simulink model "test4"  (R2021a)
settings: Solver=VariableStepAuto  StartTime=0.0  StopTime=20  RelTol=1e-1
undefined symbols (not defined in the file): B_EMB, C1, C_EMB, D_EMB, f, i_EMB, JL, JM, Jm_EMB, K1, N_EMB, rb_EMB, s_EMB, sigbuilder_block, Tc_EMB, Ts_EMB, ub_EMB
libraries: powerlib_extras x9, spsDCVoltageSourceLib x5, spsPermanentMagnetSynchronousMachineLib x5, spsUniversalBridgeLib x5, spspowerguiLib x5, spsVoltageMeasurementLib x4, pid_lib x4, simulink x3, dsparch4 x2, instrumentlib x2, Solver_SF x1
(part 3 of 3)

== matlab function test4/驱动电机模型4/2_vector_MPC_control1 ==
  settings: updateMethod=DISCRETE
  data: clock input; i_q_k input; i_d_k input; theta_e_r input; flux input; Ld input; Lq input; sa output; sb output; sc output; dtheta_e input; Te_k input; Te_ref input; phi_s_ref input
function [sa, sb, sc ] = fcn(clock, i_q_k, i_d_k, theta_e_r, flux, Ld, Lq, dtheta_e, Te_k, Te_ref, phi_s_ref)
%% 参数初始化
Ts = 0.0001;
cost = inf;
vdc = 400; % 定子电压
Rs = 0.01; % 电阻
pn = 4;
%% 获取控制周期内的相对时间
persistent time_start;
if isempty(time_start)
    time_start = clock;
end
time_relative = clock-time_start;
if time_relative >= Ts-1e-12
    time_start = clock;
    time_relative = 0;
end

%% 计算参考电压矢量
% % 无差拍控制下的phi_alpha\phi_beta
% ud_k = 0;
% ud_k = 0;
% i_d_k1 = (1-Rs*Ts/Ld)*i_d_k+Ts/Ld*(ud_k+dtheta_e*Lq*i_q_k);
% i_q_k1 = (1-Rs*Ts/Ld)*i_q_k+Ts/Ld*(uq_k-dtheta_e*Ld*i_d_k + dtheta_e*flux)

phi_dk = Ld*i_d_k +flux;
phi_qk = Lq*i_q_k;
X1 = phi_dk+dtheta_e*phi_qk*Ts;
B = ((2*Lq)/(3*pn*flux))*(Te_ref-Te_k) + (Rs*Ts*phi_qk)/Lq + dtheta_e*Ts*phi_dk;
X2 = B^2 + 2*B*(phi_qk-dtheta_e*phi_dk*Ts)+(1+dtheta_e^2*Ts^2)*(phi_dk^2+phi_qk^2) - phi_s_ref^2;
radicand = X1^2 - X2;
radicand = max(radicand, 1e-9);  % 限制最小值为1e-9，避免sqrt报错

ud_ref1 = (-X1 + sqrt(radicand)) / Ts;
ud_ref2 = (-X1 - sqrt(radicand)) / Ts;
% 选择幅值较小的解
if abs(ud_ref1) <= abs(ud_ref2)
    ud_ref = ud_ref1;
else
    ud_ref = ud_ref2;
end


uq_ref = B/Ts;
u_alpha_ref = cos(theta_e_r)*ud_ref - sin(theta_e_r)*uq_ref;
u_beta_ref = sin(theta_e_r)*ud_ref + cos(theta_e_r)*uq_ref;
theta_u_ref = atan2(u_beta_ref, u_alpha_ref);
if theta_u_ref<0
    theta_u_ref=theta_u_ref+2*pi;
end
%% 计算选择矢量
% 选择第一电压矢量
theta_norm_rel = theta_u_ref + pi/6;
if theta_norm_rel>2*pi
    theta_norm_rel=theta_norm_rel-2*pi;
end

sector = floor(theta_norm_rel / (pi/3)) + 1;
% 处理边界情况（刚好在扇区边界时归为当前扇区）
if sector == 7
    sector = 1;
end
voltage_vectors = [
    0 0 0;  % 0矢量V0
    1 0 0;  % 扇区1第一矢量V1
    1 1 0;  % 扇区2第一矢量V2
    0 1 0;  % 扇区3第一矢量V3
    0 1 1;  % 扇区4第一矢量V4
    0 0 1;  % 扇区5第一矢量V5
    1 0 1;  % 扇区6第一矢量V6
    1 1 1]; % 0矢量V7
% 选择当前扇区的第一电压矢量
first_vector = voltage_vectors(sector+1, :);
ua1 = first_vector(1)*vdc;
ub1 = first_vector(2)*vdc;
uc1 = first_vector(3)*vdc;
un1 = (ua1+ub1+uc1)/3;
u_an1 = ua1 - un1;
u_bn1 = ub1 - un1;
u_cn1 = uc1 - un1;
u_alpha_first = 2/3*(u_an1 - 1/2*u_bn1 - 1/2*u_cn1);
u_beta_first = 2/3*(sqrt(3)/2*u_bn1 - sqrt(3)/2*u_cn1);
% 选择第二电压矢量
% 开关次数约束
adjacent_sectors = {
    [7, 3, 1];  % 扇区1（V1）的相邻矢量：扇区2（V2）、扇区6（V6）
    [2, 4, 8];  % 扇区2（V2）的相邻矢量：扇区1（V1）、扇区3（V3）
    [3, 5, 1];  % 扇区3（V3）的相邻矢量：扇区2（V2）、扇区4（V4）
    [4, 6, 8];  % 扇区4（V4）的相邻矢量：扇区3（V3）、扇区5（V5）
    [5, 7, 1];  % 扇区5（V5）的相邻矢量：扇区4（V4）、扇区6（V6）
    [6, 2, 8]   % 扇区6（V6）的相邻矢量：扇区5（V5）、扇区1（V1）
    };
allowed_second_sectors = adjacent_sectors{sector};  % 允许的第二矢量sector

second_state = allowed_second_sectors(1);
for i = allowed_second_sectors
    second_vector = voltage_vectors(i,:);
    ua2 = second_vector(1)*vdc;
    ub2 = second_vector(2)*vdc;
    uc2 = second_vector(3)*vdc;
    un2 = (ua2+ub2+uc2)/3;
    u_an2 = ua2 - un2;
    u_bn2 = ub2 - un2;
    u_cn2 = uc2 - un2;
    u_alpha_second = 2/3*(u_an2 - 1/2*u_bn2 - 1/2*u_cn2);
    u_beta_second = 2/3*(sqrt(3)/2*u_bn2 - sqrt(3)/2*u_cn2);
    J = sqrt((u_alpha_ref-u_alpha_second)^2 + (u_beta_ref-u_beta_second)^2);
    if J<cost
        cost = J;
        second_state = i;
    end
    
end

second_vector = voltage_vectors(second_state, :);



%% 计算矢量作用时间
% αβ坐标系下参考电压矢量
% u_alpha_ref = Rs * i_alpha_k + (phi_alpha_k1 - phi_alpha_k)/Ts;
% u_beta_ref = Rs * i_beta_k + (phi_beta_k1 - phi_beta_k)/Ts;

% αβ坐标系下第一电压矢量
% u_alpha_first = 2/3*(u_an1 - 1/2*u_bn1 - 1/2*u_cn1);
% u_beta_first = 2/3*(sqrt(3)/2*u_bn1 - sqrt(3)/2*u_cn1);

% αβ坐标系下第二电压矢量
% u_alpha_second = 2/3*(u_an - 1/2*u_bn - 1/2*u_cn);
% u_beta_second = 2/3*(sqrt(3)/2*u_bn - sqrt(3)/2*u_cn);
num1 = (u_alpha_ref-u_alpha_second)*(u_alpha_first-u_alpha_second)+(u_beta_ref-u_beta_second)*(u_beta_first-u_beta_second);
num2 = (u_alpha_second-u_alpha_first)^2+(u_beta_second-u_beta_first)^2;
% num1 = u_alpha_ref*u_alpha_first + u_beta_ref*u_beta_first;
% num2 = u_alpha_ref^2+u_beta_ref^2;

t_1opt = num1/num2;

if t_1opt>1 
    t_1opt = 1;
end
if t_1opt<0
    t_1opt = 0;
end
% t_2opt = Ts - t_1opt;



%% 输出矢量
if time_relative < t_1opt*Ts-1e-12
%if time_relative < 2*Ts-1e-12
    sa = first_vector(1);
    sb = first_vector(2);
    sc = first_vector(3);

else
    sa = second_vector(1);
    sb = second_vector(2);
    sc = second_vector(3);    

end

== matlab function test4/驱动电机模型4/MTPA ==
  data: Te input; phi_s_ref output; Pn input; flux input; Ld input; Lq input; ita_ref output
function [phi_s_ref, ita_ref] = fcn(Te, Pn, flux, Ld, Lq)
%% MPTA原则计算phi_s_ref和ita_ref
% 对于表贴式PMSM (Ld = Lq)，MPTA条件就是id=0控制

% 计算q轴电流参考（id_ref = 0）
iq_ref = Te / (1.5 * Pn * flux);

% 计算定子磁链参考值
% phi_d = flux + Ld * id_ref = flux
% phi_q = Lq * iq_ref
phi_d_ref = flux;      % id=0
phi_q_ref = Lq * iq_ref;

phi_s_ref = sqrt(phi_d_ref^2 + phi_q_ref^2);

% 计算定子磁链参考角度
if abs(Te) < 1e-6
    ita_ref = 0;  % 零转矩时角度为0
else
    ita_ref = atan2(phi_q_ref, phi_d_ref);
end

% 确保角度在合理范围内
ita_ref = real(ita_ref);  % 避免复数
end

== matlab function test4/驱动电机模型4/phi_s_k ==
  data: id_k input; phi_s_k output; iq_k input; flux input; Ld input; Lq input; ita_k output
function [phi_s_k,ita_k]  = fcn(id_k,iq_k,flux,Ld,Lq)
phi_q_k = Lq*iq_k;
phi_d_k = Ld*id_k + flux;
phi_s_k = sqrt(phi_q_k^2+phi_d_k^2);
ita_k = atan2(phi_q_k, phi_d_k);

end

== matlab function test4/驱动电机模型1/2_vector_MPC_control1 ==
  settings: updateMethod=DISCRETE
  data: clock input; i_q_k input; i_d_k input; theta_e_r input; sa output; sb output; sc output; flux input; Ld input; Lq input; dtheta_e input; Te_k input; Te_ref input; phi_s_ref input
function [sa, sb, sc ] = fcn(clock, i_q_k, i_d_k, theta_e_r, flux, Ld, Lq, dtheta_e, Te_k, Te_ref, phi_s_ref)
%% 参数初始化
Ts = 0.0001;
cost = inf;
vdc = 400; % 定子电压
Rs = 0.11; % 电阻
pn = 4;
%% 获取控制周期内的相对时间
persistent time_start;
if isempty(time_start)
    time_start = clock;
end
time_relative = clock-time_start;
if time_relative >= Ts-1e-12
    time_start = clock;
    time_relative = 0;
end

%% 计算参考电压矢量
% % 无差拍控制下的phi_alpha\phi_beta
% ud_k = 0;
% ud_k = 0;
% i_d_k1 = (1-Rs*Ts/Ld)*i_d_k+Ts/Ld*(ud_k+dtheta_e*Lq*i_q_k);
% i_q_k1 = (1-Rs*Ts/Ld)*i_q_k+Ts/Ld*(uq_k-dtheta_e*Ld*i_d_k + dtheta_e*flux)

phi_dk = Ld*i_d_k +flux;
phi_qk = Lq*i_q_k;
X1 = phi_dk+dtheta_e*phi_qk*Ts;
B = ((2*Lq)/(3*pn*flux))*(Te_ref-Te_k) + (Rs*Ts*phi_qk)/Lq + dtheta_e*Ts*phi_dk;
X2 = B^2 + 2*B*(phi_qk-dtheta_e*phi_dk*Ts)+(1+dtheta_e^2*Ts^2)*(phi_dk^2+phi_qk^2) - phi_s_ref^2;
radicand = X1^2 - X2;
radicand = max(radicand, 1e-9);  % 限制最小值为1e-9，避免sqrt报错

ud_ref1 = (-X1 + sqrt(radicand)) / Ts;
ud_ref2 = (-X1 - sqrt(radicand)) / Ts;
% 选择幅值较小的解
if abs(ud_ref1) <= abs(ud_ref2)
    ud_ref = ud_ref1;
else
    ud_ref = ud_ref2;
end


uq_ref = B/Ts;
u_alpha_ref = cos(theta_e_r)*ud_ref - sin(theta_e_r)*uq_ref;
u_beta_ref = sin(theta_e_r)*ud_ref + cos(theta_e_r)*uq_ref;
theta_u_ref = atan2(u_beta_ref, u_alpha_ref);
if theta_u_ref<0
    theta_u_ref=theta_u_ref+2*pi;
end
%% 计算选择矢量
% 选择第一电压矢量
theta_norm_rel = theta_u_ref + pi/6;
if theta_norm_rel>2*pi
    theta_norm_rel=theta_norm_rel-2*pi;
end

sector = floor(theta_norm_rel / (pi/3)) + 1;
% 处理边界情况（刚好在扇区边界时归为当前扇区）
if sector == 7
    sector = 1;
end
voltage_vectors = [
    0 0 0;  % 0矢量V0
    1 0 0;  % 扇区1第一矢量V1
    1 1 0;  % 扇区2第一矢量V2
    0 1 0;  % 扇区3第一矢量V3
    0 1 1;  % 扇区4第一矢量V4
    0 0 1;  % 扇区5第一矢量V5
    1 0 1;  % 扇区6第一矢量V6
    1 1 1]; % 0矢量V7
% 选择当前扇区的第一电压矢量
first_vector = voltage_vectors(sector+1, :);
ua1 = first_vector(1)*vdc;
ub1 = first_vector(2)*vdc;
uc1 = first_vector(3)*vdc;
un1 = (ua1+ub1+uc1)/3;
u_an1 = ua1 - un1;
u_bn1 = ub1 - un1;
u_cn1 = uc1 - un1;
u_alpha_first = 2/3*(u_an1 - 1/2*u_bn1 - 1/2*u_cn1);
u_beta_first = 2/3*(sqrt(3)/2*u_bn1 - sqrt(3)/2*u_cn1);
% 选择第二电压矢量
% 开关次数约束
adjacent_sectors = {
    [7, 3, 1];  % 扇区1（V1）的相邻矢量：扇区2（V2）、扇区6（V6）
    [2, 4, 8];  % 扇区2（V2）的相邻矢量：扇区1（V1）、扇区3（V3）
    [3, 5, 1];  % 扇区3（V3）的相邻矢量：扇区2（V2）、扇区4（V4）
    [4, 6, 8];  % 扇区4（V4）的相邻矢量：扇区3（V3）、扇区5（V5）
    [5, 7, 1];  % 扇区5（V5）的相邻矢量：扇区4（V4）、扇区6（V6）
    [6, 2, 8]   % 扇区6（V6）的相邻矢量：扇区5（V5）、扇区1（V1）
    };
allowed_second_sectors = adjacent_sectors{sector};  % 允许的第二矢量sector

second_state = allowed_second_sectors(1);
for i = allowed_second_sectors
    second_vector = voltage_vectors(i,:);
    ua2 = second_vector(1)*vdc;
    ub2 = second_vector(2)*vdc;
    uc2 = second_vector(3)*vdc;
    un2 = (ua2+ub2+uc2)/3;
    u_an2 = ua2 - un2;
    u_bn2 = ub2 - un2;
    u_cn2 = uc2 - un2;
    u_alpha_second = 2/3*(u_an2 - 1/2*u_bn2 - 1/2*u_cn2);
    u_beta_second = 2/3*(sqrt(3)/2*u_bn2 - sqrt(3)/2*u_cn2);
    J = sqrt((u_alpha_ref-u_alpha_second)^2 + (u_beta_ref-u_beta_second)^2);
    if J<cost
        cost = J;
        second_state = i;
    end
    
end

second_vector = voltage_vectors(second_state, :);



%% 计算矢量作用时间
% αβ坐标系下参考电压矢量
% u_alpha_ref = Rs * i_alpha_k + (phi_alpha_k1 - phi_alpha_k)/Ts;
% u_beta_ref = Rs * i_beta_k + (phi_beta_k1 - phi_beta_k)/Ts;

% αβ坐标系下第一电压矢量
% u_alpha_first = 2/3*(u_an1 - 1/2*u_bn1 - 1/2*u_cn1);
% u_beta_first = 2/3*(sqrt(3)/2*u_bn1 - sqrt(3)/2*u_cn1);

% αβ坐标系下第二电压矢量
% u_alpha_second = 2/3*(u_an - 1/2*u_bn - 1/2*u_cn);
% u_beta_second = 2/3*(sqrt(3)/2*u_bn - sqrt(3)/2*u_cn);
num1 = (u_alpha_ref-u_alpha_second)*(u_alpha_first-u_alpha_second)+(u_beta_ref-u_beta_second)*(u_beta_first-u_beta_second);
num2 = (u_alpha_second-u_alpha_first)^2+(u_beta_second-u_beta_first)^2;
% num1 = u_alpha_ref*u_alpha_first + u_beta_ref*u_beta_first;
% num2 = u_alpha_ref^2+u_beta_ref^2;

t_1opt = num1/num2;

if t_1opt>1 
    t_1opt = 1;
end
if t_1opt<0
    t_1opt = 0;
end
% t_2opt = Ts - t_1opt;



%% 输出矢量
if time_relative < t_1opt*Ts-1e-12
%if time_relative < 2*Ts-1e-12
    sa = first_vector(1);
    sb = first_vector(2);
    sc = first_vector(3);

else
    sa = second_vector(1);
    sb = second_vector(2);
    sc = second_vector(3);    

end

== matlab function test4/驱动电机模型1/MTPA ==
  data: Te input; phi_s_ref output; Pn input; flux input; Ld input; Lq input; ita_ref output
function [phi_s_ref, ita_ref] = fcn(Te, Pn, flux, Ld, Lq)
%% MPTA原则计算phi_s_ref和ita_ref
% 对于表贴式PMSM (Ld = Lq)，MPTA条件就是id=0控制

% 计算q轴电流参考（id_ref = 0）
iq_ref = Te / (1.5 * Pn * flux);

% 计算定子磁链参考值
% phi_d = flux + Ld * id_ref = flux
% phi_q = Lq * iq_ref
phi_d_ref = flux;      % id=0
phi_q_ref = Lq * iq_ref;

phi_s_ref = sqrt(phi_d_ref^2 + phi_q_ref^2);

% 计算定子磁链参考角度
if abs(Te) < 1e-6
    ita_ref = 0;  % 零转矩时角度为0
else
    ita_ref = atan2(phi_q_ref, phi_d_ref);
end

% 确保角度在合理范围内
ita_ref = real(ita_ref);  % 避免复数
end

== matlab function test4/驱动电机模型1/phi_s_k ==
  data: id_k input; phi_s_k output; iq_k input; flux input; Ld input; Lq input; ita_k output
function [phi_s_k,ita_k]  = fcn(id_k,iq_k,flux,Ld,Lq)
phi_q_k = Lq*iq_k;
phi_d_k = Ld*id_k + flux;
phi_s_k = sqrt(phi_q_k^2+phi_d_k^2);
ita_k = atan2(phi_q_k, phi_d_k);

end

== matlab function test4/MPC_controller1 ==
  data: u output; thetaM_thetaL input; dthetaM_dthetaLL input; TM input; TL input; ref input
function u = mpc_controller3(thetaM_thetaL, dthetaM_dthetaLL, TM, TL, ref)
    % MPC控制器实现
    % 输入:
    %   y      - 当前系统输出
    %   r      - 参考输入(设定值)
    %   x  - 系统状态值 [dtheta1; dtheta3; dtheta2; theta1-theta2; thta1/i-theta3; TL; TM]
    %   Ts     - 采样时间
    % 输出:
    %   u      - 控制输出
    % --------------------------
    % 1. MPC参数设置
    % --------------------------
    x_hat = [thetaM_thetaL; dthetaM_dthetaLL; TM; TL];
    Np = 10;          % 预测时域
    Nc = 1;           % 控制时域
    u_min=0;
    u_max=20;
    % 设计权重矩阵
    Q = 102*eye(Np,Np);  % 状态权重矩阵
    R = 0.01;          % 控制输入权重
    Ts = 1e-5;
    %u_min = ;       % 控制输入下限
    %u_max = ;       % 控制输入上限
    %模型参数
    K1=10000;
    C1=2;
    JM=0.04;
    JL=0.1;
    i= 1;

    
    % --------------------------
    % 2. 系统模型离散化 (二阶系统)
    %    状态方程: dx/dt = Ax + Bu, y = Cx
    %    若Ts=1,离散状态方程：x(k+1)=Ts*(A+I)x(k) + Ts*Bu(k)
    % --------------------------
    A_cont = [
    0   1   0   0;                                             % 第1行
    -K1/JM-K1/JL   -C1/JM-C1/JL   1/JM  1/JL;                          % 第2行
    0  0  0  0;                                                  % 第3行
    0  0  0  0;                                                  % 第4行
    ]; % 连续时间状态矩阵
    B_cont = [0; 1/JM; 0; 0];          % 连续时间输入矩阵
    C_cont = [0 1 0 0];                % 输出矩阵
    I = eye(4,4);
    % 利用零阶保持器进行离散化
    %[A, B, C, ~] = c2d(A_cont, B_cont, C, 0, Ts);
    
    %前向欧拉法离散化
    A = Ts*A_cont+I;
    B = Ts*B_cont;
    C = C_cont;
    
    
    % --------------------------
    % 3. 构建预测模型 (状态空间形式)
    % --------------------------
    % 初始化预测矩阵
    Phi = zeros(Np*size(C,1), size(A,1));
    Gamma = zeros(Np*size(C,1), Nc);
    
    % 填充预测矩阵
    for m = 1:Np
        row_idx = (m-1)*size(C,1) + 1 : m*size(C,1);
        Phi(row_idx, :) = C*A^m;
        
        for n = 1:min(m, Nc)
            Gamma(row_idx, n) = C*A^(m-n)*B;
        end
    end
    
    % --------------------------
    % 4. 生成参考轨迹
    % --------------------------
    % 假设参考轨迹在预测时域内保持恒定
    
    
    % --------------------------
    % 5. 构建优化问题
    %    目标: min J = (Y - Y_ref)'Q_total(Y - Y_ref) + U'R_totalU
    % --------------------------
    % 构建权重矩阵
    
    
    
    
    
    % 计算跟踪误差：预测输出Y = Phi*x_hat + Gamma*U，误差 = Y - Y_ref
    Y_ref = repmat(ref, Np, 1);  % 扩展为Np×1向量（2×1）
    Y_pred = Phi * x_hat;
    
    tracking_error = Y_pred - Y_ref;  % 2x1误差向量（Np=2，n_y=1）
    
    % 修正线性项f（需转置为列向量，匹配quadprog要求）
    f = tracking_error' * Q * Gamma;  % 1xNc（Nc=1，故1x1）
    f = f';  % 转置为Nc×1列向量（1x1）
    
    % 修正二次项H（确保为Nc×Nc矩阵，R需扩展为对角矩阵）
    H = Gamma' * Q * Gamma + R * eye(Nc);  % 1x1矩阵（Nc=1）
    
    % 设置约束
    lb = repmat(u_min, Nc, 1);  % 控制输入下限
    %ub = repmat(u_max, Nc, 1);  % 控制输入上限
    
    % --------------------------
    % 6. 求解二次规划问题
    % --------------------------
    % 设置quadprog选项（指定算法为active-set）
    options = optimoptions('quadprog', ...
        'Display', 'off', ...
        'Algorithm', 'active-set', ...  % 必须指定，解决报错
        'MaxIterations', 1e3);
    % 求解优化问题
    %J_min = 0.5*U'*H*U+x_hat'*E*U;
    x0 = zeros(Nc, 1);  % Nc是控制时域，如Nc=1时x0=[0]，Nc=2时x0=[0;0]
    U = quadprog(H, f, [], [], [], [], [], [], x0, options);
    
    % --------------------------
    % 7. 应用第一个控制量 (滚动优化)
    % --------------------------
    u = U(1);
    % 防止控制量超出范围 (二次规划求解可能因数值问题略微超出)
    %u = max(min(u, u_max), u_min);
end

== matlab function test4/brake_strategy1 ==
  data: u input; y output
function y = fcn(u)

y = u;

== matlab function test4/brake_strategy ==
  data: u input; y output
function y = fcn(u)

y = u;

== matlab function test4/MATLAB Function ==
  data: reset_signal input
function stop_simulation_func(reset_signal)
% 修正版：移除了导致报错的 get_param 调用
% 功能：当接收到 Python 发来的重置信号 (1.0) 时，停止当前仿真

% 声明外部函数，告诉 Simulink 这些是 MATLAB 引擎命令，不需要生成 C 代码
coder.extrinsic('set_param');
coder.extrinsic('bdroot');
coder.extrinsic('disp');

% 阈值判断
if reset_signal > 0.5
    % 打印简单信息即可，避免复杂的字符串拼接报错
    disp('[Simulink] Received RESET signal. Stopping simulation...');
    
    % 核心命令：强制停止当前模型的仿真
    set_param(bdroot, 'SimulationCommand', 'stop');
end

end

== matlab function test4/EMB/MATLAB Function ==
  data: Fcl input; s output
function s = fcn(Fcl)

s=0;
p=[1.009081108639445e-13,-4.821675293110039e-09,1.392468214266228e-04,1.399412315201975];

% 补充物理约束：确保夹紧力非负（符合实际制动逻辑，不破坏你的格式）
if Fcl < 0
    s = 0;
end

if Fcl == 0
    s=0;
elseif Fcl<1.491117840000001e+02 && Fcl>0
    s=(Fcl+266.025)/312.603;
elseif Fcl>=1.491117840000001e+02 && Fcl<3.015520000000001e+04
    s = p(1)*Fcl^3+p(2)*Fcl^2+p(3)*Fcl^1+p(4);
elseif Fcl>=3.015520000000001e+04
    s=4;
end

s = s*1e-3;  % 保留你的相对位移计算方式
end

== matlab function test4/EMB/Subsystem1/MATLAB Function ==
  data: wm input; Tf output; Fcl input; TE input; D input; C input; Ts input; Tc input
function Tf = fcn(wm,Fcl,TE,D,C,Ts,Tc)
Tf=0;
e=10-6;

if abs(wm)>e
    Tf = D*wm+(Tc+C*Fcl)*sign(wm);
elseif abs(wm)<e && abs(TE)<(Ts+C*Fcl)
    Tf = TE;
else
    Tf = (Ts+C*Fcl)*sign(TE);
end
    
end

== matlab function test4/EMB/calculate_Fcl1/MATLAB Function ==
  data: s input; Fcl output
function Fcl = fcn(s)
s = s*1e3;  % 保留你的相对位移计算方式
Fcl =0;
% 按你的if-elseif顺序，补充s≤0的边界处理（避免Fcl未定义）
if s < 0.851 % 覆盖s≤0和0<s<0.851，均输出0（空行程/未触发）
    Fcl = 0;
elseif s >= 0.851 && s < 1.328  % 你的线性段条件
    Fcl = 312.603*s - 266.025;  % 保留你的乘法格式（标量适用）
elseif s >= 1.328 && s<=4  % 你的多项式段条件
    Fcl = -2017.2*s^3 + 16805*s^2 - 31759*s + 17412;  % 保留你的表达式
elseif s>4
    Fcl = 3.015520000000001e+04;
end

% 补充物理约束：确保夹紧力非负（符合实际制动逻辑，不破坏你的格式）
if Fcl < 0
    Fcl = 0;
end

end

== matlab function test4/EMB1/MATLAB Function ==
  data: Fcl input; s output
function s = fcn(Fcl)

s=0;
p=[1.009081108639445e-13,-4.821675293110039e-09,1.392468214266228e-04,1.399412315201975];

% 补充物理约束：确保夹紧力非负（符合实际制动逻辑，不破坏你的格式）
if Fcl < 0
    s = 0;
end

if Fcl == 0
    s=0;
elseif Fcl<1.491117840000001e+02 && Fcl>0
    s=(Fcl+266.025)/312.603;
elseif Fcl>=1.491117840000001e+02 && Fcl<3.015520000000001e+04
    s = p(1)*Fcl^3+p(2)*Fcl^2+p(3)*Fcl^1+p(4);
elseif Fcl>=3.015520000000001e+04
    s=4;
end

s = s*1e-3;  % 保留你的相对位移计算方式
end

== matlab function test4/EMB1/Subsystem1/MATLAB Function ==
  data: wm input; Tf output; Fcl input; TE input; D input; C input; Ts input; Tc input
function Tf = fcn(wm,Fcl,TE,D,C,Ts,Tc)
Tf=0;
e=10-6;

if abs(wm)>e
    Tf = D*wm+(Tc+C*Fcl)*sign(wm);
elseif abs(wm)<e && abs(TE)<(Ts+C*Fcl)
    Tf = TE;
else
    Tf = (Ts+C*Fcl)*sign(TE);
end
    
end
